simulink subsystem "GravityGradient_SS"  (R2023a)
settings: Solver=VariableStepAuto  StartTime=0.0  StopTime=10.0  RelTol=1e-3
settings Model: Creator=jself  LastModifiedBy=jself

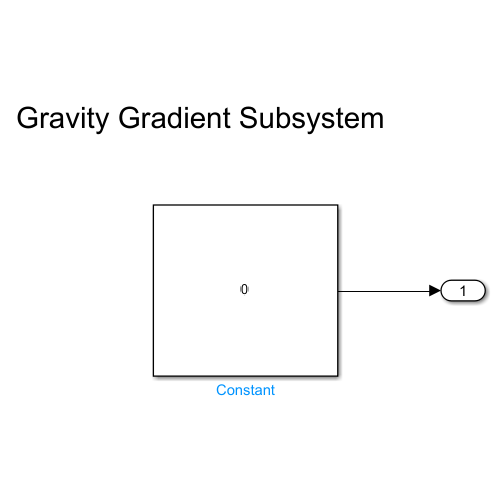
[thumbnail: Simulink's stored preview of the top-level diagram]
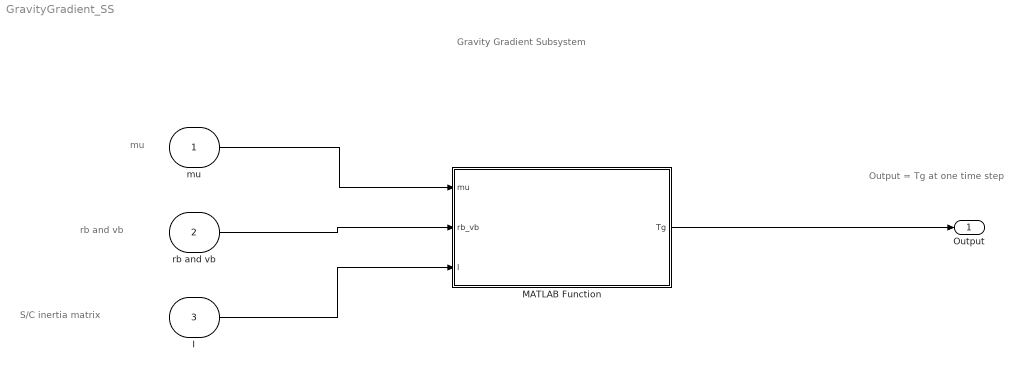
== system GravityGradient_SS ==
  note: Output = Tg at one time step
  note: Gravity Gradient Subsystem
  note: mu
  note: rb and vb
  note: S/C inertia matrix
  mu : Inport
  rb and vb : Inport  Port=2
  I : Inport  Port=3
  MATLAB Function : MATLAB Function  TreatAsAtomicUnit=on
  Output : Outport
  wires:
  mu/1 -> MATLAB Function/1(mu)
  rb and vb/1 -> MATLAB Function/2(rb_vb)
  I/1 -> MATLAB Function/3(I)
  MATLAB Function/1(Tg) -> Output/1

== matlab function GravityGradient_SS/MATLAB Function ==
  data: mu input; Tg output; rb_vb input; I input
function Tg = gravgradient(mu,rb_vb,I)

%{
INPUTS: 
        mu = grav parameter of central body
        r = spacecraft position vector in BODY coordinates
        I = inertia matrix of the s/c
    Author: Justin Self
    May 19, 2023
%}

rb = rb_vb(1:3);

rb_cross = [     0       -rb(3)     rb(2);
                rb(3)    0         -rb(1);
               -rb(2)    rb(1)       0   ];

Tg = ( (3*mu) / (norm(rb)^5) ) * (rb_cross * I * rb); 


% CHECKS
% 3x1; good
% units are in J or N*m; OK

end
